simulink model "deliverable2"  (R2020a)
settings: Solver=FixedStepAuto  StartTime=0.0  StopTime=10.0  FixedStep=1e-3  RelTol=1e-3  EnableMultiTasking=on
undefined symbols (not defined in the file): A0, A1, D0, D1, D10, D11, D12, D13, D2, D3, D4, D5, D6, D7, D8, D9, PTA0, PTA1, PTA2, PTB2, PTB23, PTB3, PTB9, PTC16, PTC17, PTC2, PTC3, PTC4, PTD0, PTD1, PTD2, PTD3
libraries: frdmk64flib x21, simulink x3, etargetslib x2
settings Model: ExtModeTrigDuration=5  Creator=Abrar Hussain  LastModifiedBy=Nabil
settings SolverCC: AutoInsertRateTranBlk=on
settings OptimizationCC: EnhancedBackFolding=on  PassReuseOutputArgsAs=Individual arguments  ZeroExternalMemoryAtStartup=off  ZeroInternalMemoryAtStartup=off  MaxStackSize=64  OptimizeBlockOrder=speed  DifferentSizesBufferReuse=on  OptimizationCustomize=off  EfficientTunableParamExpr=on
settings DebuggingCC: ParameterTunabilityLossMsg=error
settings HardwareCC: ProdBitPerPointer=32  ProdBitPerSizeT=32  ProdBitPerPtrDiffT=32  ProdLargestAtomicInteger=Long  ProdLargestAtomicFloat=Double  ProdWordSize=32  ProdHWDeviceType=ARM Compatible->ARM Cortex
settings SFSimCC: MATLABDynamicMemAlloc=off
settings RTWCC: SystemTargetFile=ert.tlc  HardwareBoard=NXP FRDM-K64F  TemplateMakefile=ert_default_tmf  Toolchain=GNU Tools for ARM Embedded Processors
settings CodeAppCC: ForceParamTrailComments=on  IgnoreCustomStorageClasses=off  OperatorAnnotations=on  SimulinkDataObjDesc=on  SFDataObjDesc=on  InsertBlockDesc=on

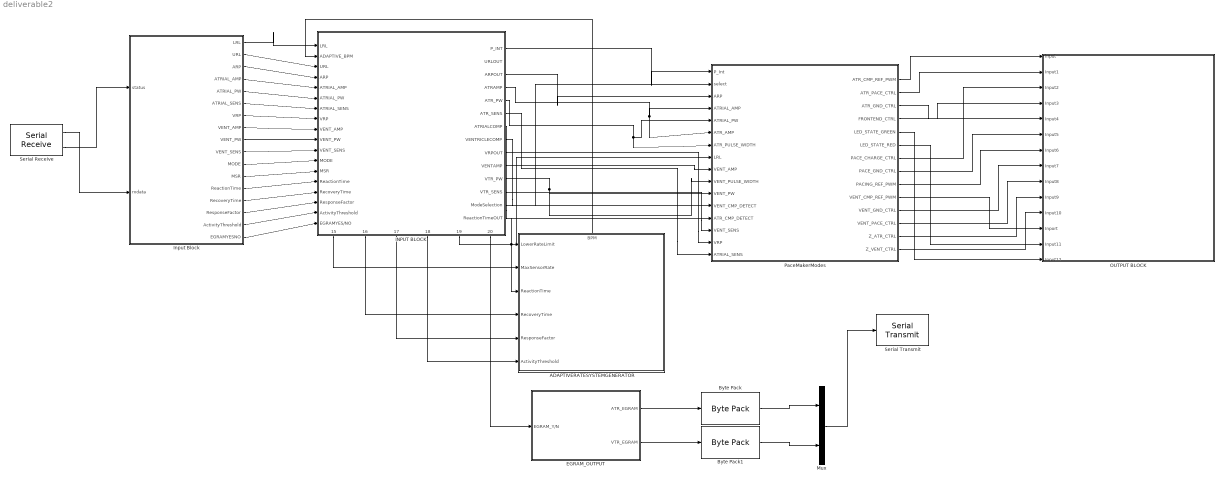
== system deliverable2 ==
  ADAPTIVERATESYSTEMGENERATOR : Subsystem
      settings: PortSchema="{\"entries\":[{\"content\":{\"sides\":[{\"content\":{\"connectorIds\":[\"In1\",\"In2\",\"In3\",\"In4\",\"In5\",\"In6\"]},\"type\":\"ConnectorPlacement.EquallySpacedRectSide\",\"uuid\":\"97e3620a-bd9c-448b-97fc-3b1c936c5d8f\"},{\"content\":{\"connectorIds\":[],\"side\":\"RIGHT\"},\"type\":\"ConnectorPlacement.EquallySpacedRectSide\",\"uuid\":\"57bdd7e3-75eb-4ddf-876e-8d78bd49943e\"},{\"content\":{\"connectorIds\":[\"Out1\"],\"side\":\"TOP\"},\"type\":\"ConnectorPlacement.EquallySpacedRectSide\",\"uuid\":\"a5076879-9988-488c-a84d-5198dc545756\"}]},\"type\":\"ConnectorPlacement.EquallySpacedConnector\",\"uuid\":\"f48a9ccb-b26f-4eb4-a375-26685a890dd7\"}],\"packageUris\":[\"http://schema.mathworks.com/mf0/Connector/19700101\"],\"version\":\"1.0\"}"
  Byte Pack : etargetslib/Byte Pack  datatypes={'double'}  byteAlign=1
  Byte Pack1 : etargetslib/Byte Pack  datatypes={'double'}  byteAlign=1
  EGRAM_OUTPUT : Subsystem
  INPUT BLOCK : Subsystem
      settings: PortSchema="{\"entries\":[{\"content\":{\"sides\":[{\"content\":{\"connectorIds\":[\"In1\",\"In2\",\"In3\",\"In4\",\"In5\",\"In6\",\"In7\",\"In8\",\"In9\",\"In10\",\"In11\",\"In12\",\"In13\",\"In14\",\"In15\",\"In16\",\"In17\",\"In18\"]},\"type\":\"ConnectorPlacement.EquallySpacedRectSide\",\"uuid\":\"b7991482-aae8-494c-b95e-38f3914ca862\"},{\"content\":{\"connectorIds\":[\"Out1\",\"Out2\",\"Out3\",\"Out4\",\"Out5\",\"Out6\",\"Out7\",\"Out8\",\"Out9\",\"Out10\",\"Out11\",\"Out12\",\"Out13\",\"Out14\"],\"side\":\"RIGHT\"},\"type\":\"ConnectorPlacement.EquallySpacedRectSide\",\"uuid\":\"a5db160a-6579-43b0-bce8-09045d3fe5a5\"},{\"content\":{\"connectorIds\":[],\"side\":\"TOP\"},\"type\":\"ConnectorPlacement.EquallySpacedRectSide\",\"uuid\":\"59d47d4e-9fe5-4943-8fba-05eb32ac822f\"},{\"content\":{\"connectorIds\":[\"Out15\",\"Out16\",\"Out17\",\"Out18\",\"Out19\",\"Out20\"],\"side\":\"BOTTOM\"},\"type\":\"ConnectorPlacement.EquallySpacedRectSide\",\"uuid\":\"ee0852ae-153e-4381-9b18-f12d1b0cb66f\"}]},\"type\":\"ConnectorPlacement.EquallySpacedConnector\",\"uuid\":\"9fb077cb-2923-469d-be1e-c13020122ede\"}],\"packageUris\":[\"http://schema.mathworks.com/mf0/Connector/19700101\"],\"version\":\"1.0\"}"
  Input Block : Stateflow chart  TreatAsAtomicUnit=on
  Mux : Mux  Inputs=2
  OUTPUT BLOCK : Subsystem
  PaceMakerModes : Stateflow chart  TreatAsAtomicUnit=on
      settings: PortSchema="{\"entries\":[{\"content\":{\"sides\":[{\"content\":{\"connectorIds\":[\"In1\",\"In2\",\"In3\",\"In4\",\"In5\",\"In6\",\"In7\",\"In8\",\"In9\",\"In10\",\"In11\",\"In12\",\"In13\",\"In14\",\"In15\",\"In16\"]},\"type\":\"ConnectorPlacement.EquallySpacedRectSide\",\"uuid\":\"26878569-42a4-4c6e-8e2e-b0c46cc4aa32\"},{\"content\":{\"connectorIds\":[\"Out1\",\"Out3\",\"Out2\",\"Out4\",\"Out5\",\"Out6\",\"Out7\",\"Out8\",\"Out9\",\"Out10\",\"Out11\",\"Out12\",\"Out13\",\"Out14\"],\"side\":\"RIGHT\"},\"type\":\"ConnectorPlacement.EquallySpacedRectSide\",\"uuid\":\"54e40a9a-b8cb-48bd-a159-657a41086fa1\"},{\"content\":{\"connectorIds\":[],\"side\":\"TOP\"},\"type\":\"ConnectorPlacement.EquallySpacedRectSide\",\"uuid\":\"729d6bf4-f6e0-4315-bd55-b919cf68ae5a\"}]},\"type\":\"ConnectorPlacement.EquallySpacedConnector\",\"uuid\":\"8ffc528b-0e13-4f9b-b36d-bd07e577bd5a\"}],\"packageUris\":[\"http://schema.mathworks.com/mf0/Connector/19700101\"],\"version\":\"1.0\"}"
  Serial Receive : frdmk64flib/Serial Receive  SCIModule=0  Baudrate=uint32(9600)  Parity=None  StopBits=1  HardwareFlowControl=None  ByteOrder=LittleEndian  DataType=uint8  DataLength=20  BlockingMode=off  OutputStatus=on  SampleTime=0.1
  Serial Transmit : frdmk64flib/Serial Transmit  SCIModule=0  Baudrate=uint32(9600)  Parity=None  StopBits=1  HardwareFlowControl=None  ByteOrder=LittleEndian  BlockingMode=on  OutputStatus=off
  wires:
  INPUT BLOCK/20(EGRAMBUTTON) -> EGRAM_OUTPUT/1(EGRAM_Y/N)
  EGRAM_OUTPUT/1(ATR_EGRAM) -> Byte Pack/1
  EGRAM_OUTPUT/2(VTR_EGRAM) -> Byte Pack1/1
  ADAPTIVERATESYSTEMGENERATOR/1(BPM) -> INPUT BLOCK/2(ADAPTIVE_BPM)
  INPUT BLOCK/19(LowerRateLimit) -> PaceMakerModes/8(LRL), ADAPTIVERATESYSTEMGENERATOR/1(LowerRateLimit)
  INPUT BLOCK/15(MaxSensorRate) -> ADAPTIVERATESYSTEMGENERATOR/2(MaxSensorRate)
  INPUT BLOCK/14(ReactionTimeOUT) -> ADAPTIVERATESYSTEMGENERATOR/3(ReactionTime)
  INPUT BLOCK/16(RecoveryTimeOUT) -> ADAPTIVERATESYSTEMGENERATOR/4(RecoveryTime)
  INPUT BLOCK/17(ResponseFactorOUT) -> ADAPTIVERATESYSTEMGENERATOR/5(ResponseFactor)
  INPUT BLOCK/18(ActivityThresholdOUT) -> ADAPTIVERATESYSTEMGENERATOR/6(ActivityThreshold)
  INPUT BLOCK/1(P_INT) -> PaceMakerModes/1(P_Int)
  INPUT BLOCK/3(ARPOUT) -> PaceMakerModes/3(ARP)
  INPUT BLOCK/13(ModeSelection) -> PaceMakerModes/2(select)
  INPUT BLOCK/4(ATRAMP) -> PaceMakerModes/6(ATR_AMP), PaceMakerModes/4(ATRIAL_AMP)
  INPUT BLOCK/5(ATR_PW) -> PaceMakerModes/7(ATR_PULSE_WIDTH), PaceMakerModes/5(ATRIAL_PW)
  INPUT BLOCK/6(ATR_SENS) -> PaceMakerModes/16(ATRIAL_SENS)
  INPUT BLOCK/7(ATRIALCOMP) -> PaceMakerModes/13(ATR_CMP_DETECT)
  INPUT BLOCK/8(VENTRICLECOMP) -> PaceMakerModes/12(VENT_CMP_DETECT)
  INPUT BLOCK/9(VRPOUT) -> PaceMakerModes/15(VRP)
  INPUT BLOCK/10(VENTAMP) -> PaceMakerModes/9(VENT_AMP)
  INPUT BLOCK/11(VTR_PW) -> PaceMakerModes/10(VENT_PULSE_WIDTH), PaceMakerModes/11(VENT_PW)
  INPUT BLOCK/12(VTR_SENS) -> PaceMakerModes/14(VENT_SENS)
  PaceMakerModes/1(ATR_CMP_REF_PWM) -> OUTPUT BLOCK/1(Input)
  PaceMakerModes/3(ATR_PACE_CTRL) -> OUTPUT BLOCK/2(Input1)
  PaceMakerModes/7(PACE_CHARGE_CTRL) -> OUTPUT BLOCK/3(Input2)
  PaceMakerModes/4(FRONTEND_CTRL) -> OUTPUT BLOCK/4(Input3)
  PaceMakerModes/2(ATR_GND_CTRL) -> OUTPUT BLOCK/5(Input4)
  PaceMakerModes/8(PACE_GND_CTRL) -> OUTPUT BLOCK/6(Input5)
  PaceMakerModes/9(PACING_REF_PWM) -> OUTPUT BLOCK/7(Input6)
  PaceMakerModes/14(Z_VENT_CTRL) -> OUTPUT BLOCK/11(Input10)
  PaceMakerModes/13(Z_ATR_CTRL) -> OUTPUT BLOCK/10(Input9)
  PaceMakerModes/12(VENT_PACE_CTRL) -> OUTPUT BLOCK/9(Input8)
  PaceMakerModes/11(VENT_GND_CTRL) -> OUTPUT BLOCK/8(Input7)
  PaceMakerModes/10(VENT_CMP_REF_PWM) -> OUTPUT BLOCK/12(Inport)
  PaceMakerModes/6(LED_STATE_RED) -> OUTPUT BLOCK/13(Input11)
  PaceMakerModes/5(LED_STATE_GREEN) -> OUTPUT BLOCK/14(Input12)
  Input Block/1(LRL) -> INPUT BLOCK/1("LRL ")
  Input Block/2(URL) -> INPUT BLOCK/3(URL)
  Input Block/3(ARP) -> INPUT BLOCK/4(ARP)
  Input Block/4(ATRIAL_AMP) -> INPUT BLOCK/5(ATRIAL_AMP)
  Input Block/5(ATRIAL_PW) -> INPUT BLOCK/6(ATRIAL_PW)
  Input Block/6(ATRIAL_SENS) -> INPUT BLOCK/7(ATRIAL_SENS)
  Input Block/7(VRP) -> INPUT BLOCK/8(VRP)
  Input Block/8(VENT_AMP) -> INPUT BLOCK/9(VENT_AMP)
  Input Block/9(VENT_PW) -> INPUT BLOCK/10(VENT_PW)
  Input Block/10(VENT_SENS) -> INPUT BLOCK/11(VENT_SENS)
  Input Block/11(MODE) -> INPUT BLOCK/12(MODE)
  Input Block/12(MSR) -> INPUT BLOCK/13(MSR)
  Input Block/13(ReactionTime) -> INPUT BLOCK/14(ReactionTime)
  Input Block/14(RecoveryTime) -> INPUT BLOCK/15(RecoveryTime)
  Input Block/15(ResponseFactor) -> INPUT BLOCK/16(ResponseFactor)
  Input Block/16(ActivityThreshold) -> INPUT BLOCK/17(ActivityThreshold)
  Input Block/17(EGRAMYESNO) -> INPUT BLOCK/18(EGRAMYES/NO)
  Serial Receive/2 -> Input Block/1(status)
  Serial Receive/1 -> Input Block/2(rxdata)
  Byte Pack/1 -> Mux/1
  Byte Pack1/1 -> Mux/2
  Mux/1 -> Serial Transmit/1

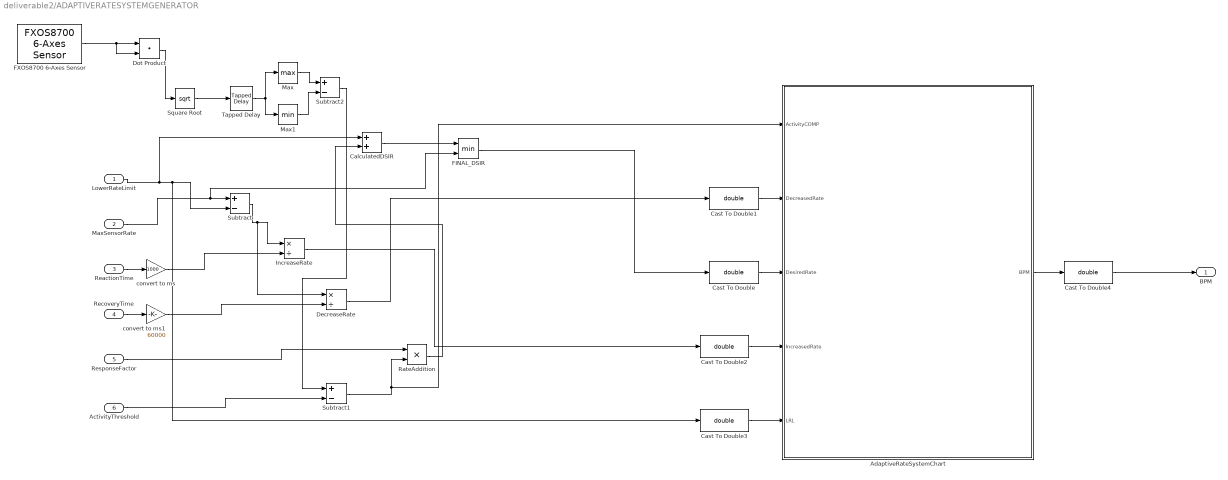
== system deliverable2/ADAPTIVERATESYSTEMGENERATOR ==
  LowerRateLimit : Inport
  MaxSensorRate : Inport  Port=2
  ReactionTime : Inport  Port=3
  RecoveryTime : Inport  Port=4
  ResponseFactor : Inport  Port=5
  ActivityThreshold : Inport  Port=6
  AdaptiveRateSystemChart : Stateflow chart  TreatAsAtomicUnit=on
  CalculatedDSIR : Sum
  Cast To Double{,1..4} (5 alike) : DataTypeConversion  OutDataTypeStr=double
  DecreaseRate : Product  Inputs=*/
  Dot Product : DotProduct  RndMeth=Nearest  InputSameDT=on  OutDataTypeStr=Inherit: Inherit via internal rule
  FINAL_DSIR : MinMax  Inputs=2
  FXOS8700 6-Axes Sensor : frdmk64flib/FXOS8700 6-Axes Sensor  Activesensor=Accelerometer only  ODR=800Hz  HybridODR=400Hz  Accelfullrange=-4g to +4g  SampleTime=-1
  IncreaseRate : Product  Inputs=*/
  Max : MinMax  Function=max
  Max1 : MinMax
  RateAddition : Product
  Square Root : Sqrt  SaturateOnIntegerOverflow=on
  Subtract : Sum  Inputs=+-
  Subtract1 : Sum  Inputs=+-
  Subtract2 : Sum  Inputs=+-
  Tapped Delay : simulink/Discrete/Tapped Delay  vinit=0.0  samptime=0.002  NumDelays=99  DelayOrder=Oldest  includeCurrent=on
  convert to ms : Gain  Gain=1000
  convert to ms1 : Gain  Gain=60000
  BPM : Outport
  wires:
  LowerRateLimit/1 -> CalculatedDSIR/1, Cast To Double3/1, Subtract/2
  Subtract/1 -> DecreaseRate/1, IncreaseRate/1
  ReactionTime/1 -> convert to ms/1
  RecoveryTime/1 -> convert to ms1/1
  ActivityThreshold/1 -> Subtract1/2
  Subtract2/1 -> Subtract1/1
  ResponseFactor/1 -> RateAddition/1
  RateAddition/1 -> CalculatedDSIR/2
  CalculatedDSIR/1 -> FINAL_DSIR/1
  MaxSensorRate/1 -> FINAL_DSIR/2, Subtract/1
  FINAL_DSIR/1 -> Cast To Double/1
  IncreaseRate/1 -> Cast To Double2/1
  DecreaseRate/1 -> Cast To Double1/1
  AdaptiveRateSystemChart/1(BPM) -> Cast To Double4/1
  Subtract1/1 -> AdaptiveRateSystemChart/1(ActivityCOMP), RateAddition/2
  Cast To Double1/1 -> AdaptiveRateSystemChart/2(DecreasedRate)
  Cast To Double/1 -> AdaptiveRateSystemChart/3(DesiredRate)
  Cast To Double2/1 -> AdaptiveRateSystemChart/4(IncreasedRate)
  Cast To Double3/1 -> AdaptiveRateSystemChart/5(LRL)
  Cast To Double4/1 -> BPM/1
  convert to ms/1 -> IncreaseRate/2
  convert to ms1/1 -> DecreaseRate/2
  Tapped Delay/1 -> Max/1, Max1/1
  Max1/1 -> Subtract2/2
  FXOS8700 6-Axes Sensor/1 -> Dot Product/2, Dot Product/1
  Max/1 -> Subtract2/1
  Square Root/1 -> Tapped Delay/1
  Dot Product/1 -> Square Root/1

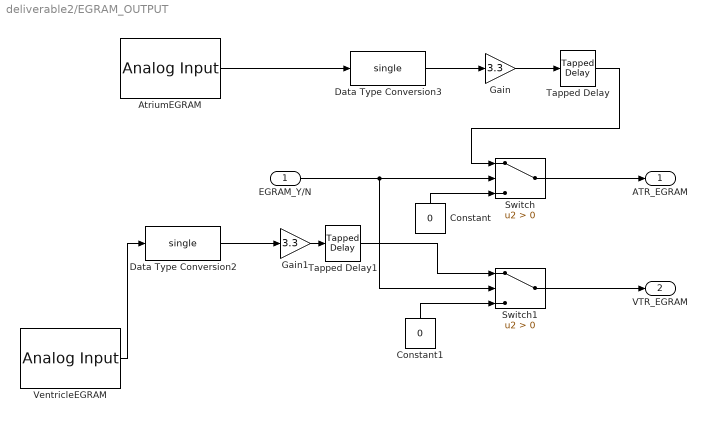
== system deliverable2/EGRAM_OUTPUT ==
  EGRAM_Y/N : Inport
  AtriumEGRAM : frdmk64flib/Analog Input  Whichpin=PTB2 (A0)  SampleTime=-1
  Constant : Constant  Value=0
  Constant1 : Constant  Value=0
  Data Type Conversion2 : DataTypeConversion  OutDataTypeStr=single  RndMeth=Nearest
  Data Type Conversion3 : DataTypeConversion  OutDataTypeStr=single  RndMeth=Nearest
  Gain : Gain  Gain=3.3
  Gain1 : Gain  Gain=3.3
  Switch : Switch  Criteria=u2 > Threshold
  Switch1 : Switch  Criteria=u2 > Threshold
  Tapped Delay : simulink/Discrete/Tapped Delay  vinit=0.0  samptime=0.002  NumDelays=9  DelayOrder=Oldest  includeCurrent=on
  Tapped Delay1 : simulink/Discrete/Tapped Delay  vinit=0.0  samptime=0.002  NumDelays=9  DelayOrder=Oldest  includeCurrent=on
  VentricleEGRAM : frdmk64flib/Analog Input  Whichpin=PTB3 (A1)  SampleTime=-1
  ATR_EGRAM : Outport
  VTR_EGRAM : Outport  Port=2
  wires:
  EGRAM_Y/N/1 -> Switch1/2, Switch/2
  Switch/1 -> ATR_EGRAM/1
  Switch1/1 -> VTR_EGRAM/1
  Data Type Conversion3/1 -> Gain/1
  Gain1/1 -> Tapped Delay1/1
  VentricleEGRAM/1 -> Data Type Conversion2/1
  Tapped Delay1/1 -> Switch1/1
  Tapped Delay/1 -> Switch/1
  AtriumEGRAM/1 -> Data Type Conversion3/1
  Gain/1 -> Tapped Delay/1
  Data Type Conversion2/1 -> Gain1/1
  Constant/1 -> Switch/3
  Constant1/1 -> Switch1/3

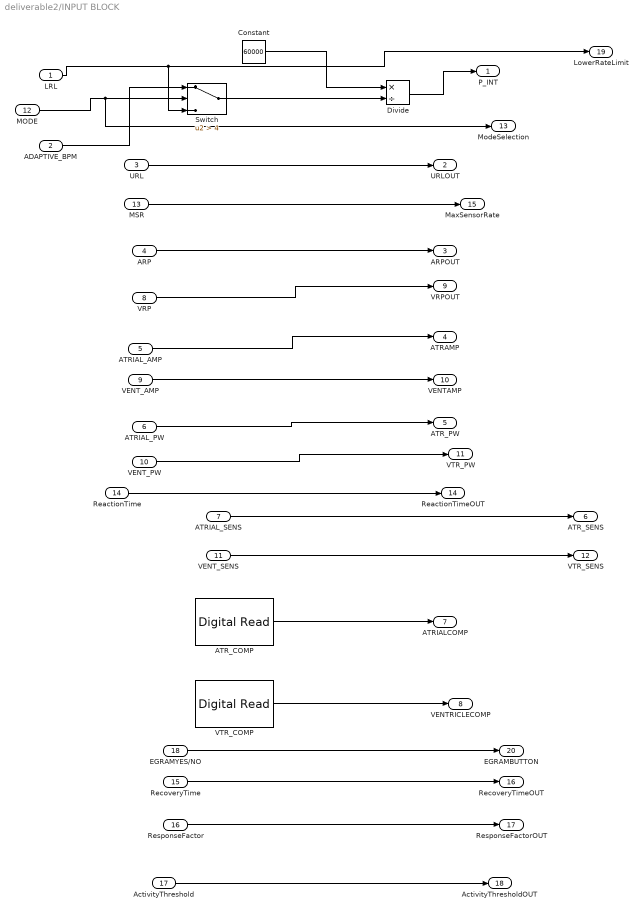
== system deliverable2/INPUT BLOCK ==
  "LRL " : Inport
  ADAPTIVE_BPM : Inport  Port=2
  URL : Inport  Port=3
  ARP : Inport  Port=4
  ATRIAL_AMP : Inport  Port=5
  ATRIAL_PW : Inport  Port=6
  ATRIAL_SENS : Inport  Port=7
  VRP : Inport  Port=8
  VENT_AMP : Inport  Port=9
  VENT_PW : Inport  Port=10
  VENT_SENS : Inport  Port=11
  MODE : Inport  Port=12
  MSR : Inport  Port=13
  ReactionTime : Inport  Port=14
  RecoveryTime : Inport  Port=15
  ResponseFactor : Inport  Port=16
  ActivityThreshold : Inport  Port=17
  EGRAMYES/NO : Inport  Port=18
  ATR_COMP : frdmk64flib/Digital Read  Whichpin=PTC16 (D0)  SampleTime=-1
  Constant : Constant  Value=60000
  Divide : Product  Inputs=*/
  Switch : Switch  Criteria=u2 > Threshold  Threshold=4
  VTR_COMP : frdmk64flib/Digital Read  Whichpin=PTC17 (D1)  SampleTime=-1
  P_INT : Outport
  URLOUT : Outport  Port=2
  ARPOUT : Outport  Port=3
  ATRAMP : Outport  Port=4
  ATR_PW : Outport  Port=5
  ATR_SENS : Outport  Port=6
  ATRIALCOMP : Outport  Port=7
  VENTRICLECOMP : Outport  Port=8
  VRPOUT : Outport  Port=9
  VENTAMP : Outport  Port=10
  VTR_PW : Outport  Port=11
  VTR_SENS : Outport  Port=12
  ModeSelection : Outport  Port=13
  ReactionTimeOUT : Outport  Port=14
  MaxSensorRate : Outport  Port=15
  RecoveryTimeOUT : Outport  Port=16
  ResponseFactorOUT : Outport  Port=17
  ActivityThresholdOUT : Outport  Port=18
  LowerRateLimit : Outport  Port=19
  EGRAMBUTTON : Outport  Port=20
  wires:
  URL/1 -> URLOUT/1
  ARP/1 -> ARPOUT/1
  ATR_COMP/1 -> ATRIALCOMP/1
  ATRIAL_AMP/1 -> ATRAMP/1
  ATRIAL_PW/1 -> ATR_PW/1
  ATRIAL_SENS/1 -> ATR_SENS/1
  Constant/1 -> Divide/1
  Divide/1 -> P_INT/1
  Switch/1 -> Divide/2
  "LRL "/1 -> LowerRateLimit/1, Switch/3
  ADAPTIVE_BPM/1 -> Switch/1
  VTR_COMP/1 -> VENTRICLECOMP/1
  VRP/1 -> VRPOUT/1
  VENT_AMP/1 -> VENTAMP/1
  VENT_PW/1 -> VTR_PW/1
  VENT_SENS/1 -> VTR_SENS/1
  MODE/1 -> ModeSelection/1, Switch/2
  MSR/1 -> MaxSensorRate/1
  ReactionTime/1 -> ReactionTimeOUT/1
  RecoveryTime/1 -> RecoveryTimeOUT/1
  ResponseFactor/1 -> ResponseFactorOUT/1
  ActivityThreshold/1 -> ActivityThresholdOUT/1
  EGRAMYES/NO/1 -> EGRAMBUTTON/1

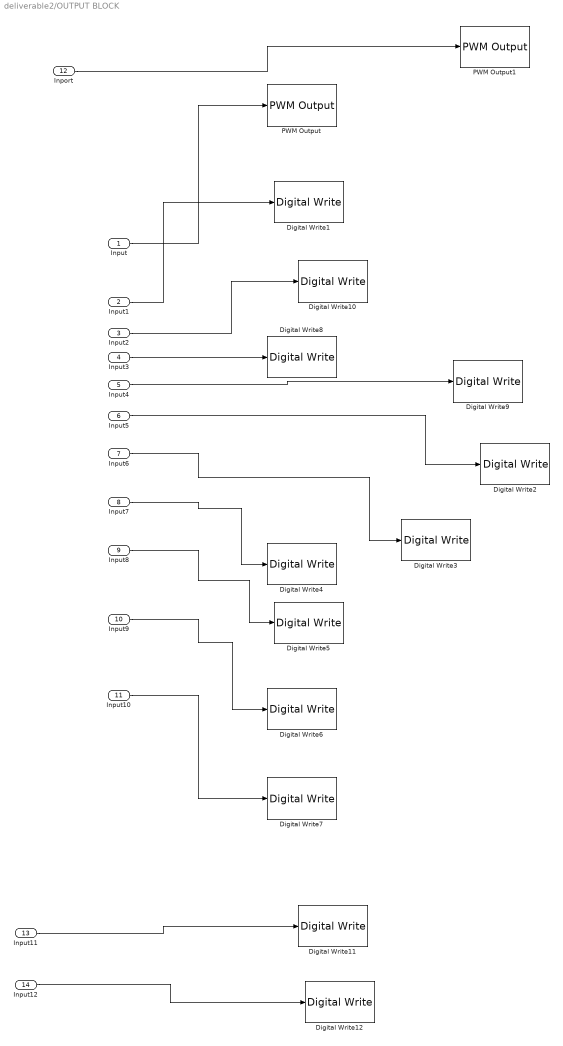
== system deliverable2/OUTPUT BLOCK ==
  Input : Inport
  Input1 : Inport  Port=2
  Input2 : Inport  Port=3
  Input3 : Inport  Port=4
  Input4 : Inport  Port=5
  Input5 : Inport  Port=6
  Input6 : Inport  Port=7
  Input7 : Inport  Port=8
  Input8 : Inport  Port=9
  Input9 : Inport  Port=10
  Input10 : Inport  Port=11
  Inport : Inport  Port=12
  Input11 : Inport  Port=13
  Input12 : Inport  Port=14
  Digital Write1 : frdmk64flib/Digital Write  Whichpin=PTA0 (D8)
  Digital Write10 : frdmk64flib/Digital Write  Whichpin=PTB9 (D2)
  Digital Write11 : frdmk64flib/Digital Write  Whichpin=RED_LED
  Digital Write12 : frdmk64flib/Digital Write  Whichpin=GREEN_LED
  Digital Write2 : frdmk64flib/Digital Write  Whichpin=PTD0 (D10)
  Digital Write3 : frdmk64flib/Digital Write  Whichpin=PTA2 (D5)
  Digital Write4 : frdmk64flib/Digital Write  Whichpin=PTD3 (D12)
  Digital Write5 : frdmk64flib/Digital Write  Whichpin=PTC4 (D9)
  Digital Write6 : frdmk64flib/Digital Write  Whichpin=PTB23 (D4)
  Digital Write7 : frdmk64flib/Digital Write  Whichpin=PTC3 (D7)
  Digital Write8 : frdmk64flib/Digital Write  Whichpin=PTD1 (D13)
  Digital Write9 : frdmk64flib/Digital Write  Whichpin=PTD2 (D11)
  PWM Output : frdmk64flib/PWM Output  Whichpin=PTC2 (D6)  InitialFrequency=2000  InitialDutyCycle=0
  PWM Output1 : frdmk64flib/PWM Output  Whichpin=PTA1 (D3)  InitialFrequency=2000  InitialDutyCycle=0
  wires:
  Input/1 -> PWM Output/1
  Input1/1 -> Digital Write1/1
  Input10/1 -> Digital Write7/1
  Input9/1 -> Digital Write6/1
  Input8/1 -> Digital Write5/1
  Input7/1 -> Digital Write4/1
  Input6/1 -> Digital Write3/1
  Input5/1 -> Digital Write2/1
  Input4/1 -> Digital Write9/1
  Input3/1 -> Digital Write8/1
  Input2/1 -> Digital Write10/1
  Inport/1 -> PWM Output1/1
  Input11/1 -> Digital Write11/1
  Input12/1 -> Digital Write12/1

== stateflow chart deliverable2/ADAPTIVERATESYSTEMGENERATOR/AdaptiveRateSystemChart ==
  state PowerOnReset
    entry:
    BPM = LRL;
    elapsed_time = 0;
  state ActivityGreaterDecrease
    entry:
    elapsed_time = elapsed(msec);
    BPM = BPM - (DecreasedRate*elapsed_time);
  state ActivitySmallerDecrease
    entry:
    elapsed_time = elapsed(msec);
    BPM = BPM - (DecreasedRate*elapsed_time);
  state CheckActivity
  state ActivityGreaterIncrease
    entry:
    elapsed_time = elapsed(msec);
    BPM = BPM + (IncreasedRate*elapsed_time);
  state DesiredRateMet
    entry:
    elapsed_time = 0;
    BPM = DesiredRate;
  state LowerRateMet
    entry:
    BPM = LRL;
    elapsed_time = 0;
  (default) -> PowerOnReset
  PowerOnReset -> CheckActivity
  (junction 13) -> ActivityGreaterDecrease [order 1] : [DesiredRate < BPM]
  ActivityGreaterDecrease -> DesiredRateMet : [BPM <= DesiredRate]
  CheckActivity -> (junction 13) [order 1] : [ActivityCOMP  > 0]
  CheckActivity -> (junction 30) [order 2] : [ActivityCOMP <= 0]
  (junction 13) -> ActivityGreaterIncrease [order 2] : [DesiredRate > BPM]
  (junction 13) -> DesiredRateMet [order 3] : [BPM == DesiredRate]
  (junction 30) -> ActivitySmallerDecrease [order 2] : [BPM  >= LRL]
  (junction 30) -> LowerRateMet [order 1] : [BPM == LRL]
  (junction 27) -> CheckActivity : [after(60/BPM,sec)]
  ActivitySmallerDecrease -> LowerRateMet : [BPM <= LRL]
  DesiredRateMet -> (junction 27)
  LowerRateMet -> (junction 27)
  ActivityGreaterIncrease -> DesiredRateMet : [BPM >= DesiredRate]
  data: BPM output; ActivityCOMP input; DecreasedRate input; DesiredRate input; IncreasedRate input; LRL input; elapsed_time local

== stateflow chart deliverable2/Input Block ==
  state Set_param
    entry:
    LRL = cast(rxdata(3),'uint16');
    URL = cast(rxdata(4),'uint16');
    ARP = cast(rxdata(5),'uint16');
    ATRIAL_AMP = cast(rxdata(6),'double');
    ATRIAL_PW = cast(rxdata(7),'uint16');
    ATRIAL_SENS = cast(rxdata(8),'double');
    VRP = cast(rxdata(9),'uint16');
    VENT_AMP = cast(rxdata(10),'double');
    VENT_PW = cast(rxdata(11),'double');
    VENT_SENS = cast(rxdata(12),'double');
    MODE = cast(rxdata(13),'uint16');
    MSR = cast(rxdata(14),'uint16');
    ReactionTime = cast(rxdata(15),'uint16');
    RecoveryTime = cast(rxdata(16),'uint16');
    ResponseFactor = cast(rxdata(17),'double');
    ActivityThreshold = cast(rxdata(18),'double');
    EGRAMYESNO = cast(rxdata(19),'uint16');
  state Initial
    entry:
    LRL = 60;
    URL = 120;
    ARP = 250;
    ATRIAL_AMP = 3.75;
    ATRIAL_PW = 0;
    ATRIAL_SENS = 0.75;
    VRP = 320;
    VENT_AMP = 3.75;
    VENT_PW = 0;
    VENT_SENS = 2.5;
    MODE = 5;
    MSR = 120;
    ReactionTime = 30;
    RecoveryTime = 5;
    ResponseFactor = 8;
    ActivityThreshold = 30;
    EGRAMYESNO = 0;
  state Standby
    %waiting for COM
  (default) -> Initial
  Set_param -> Standby
  (junction 62) -> ? : [rxdata(2)==hex2dec('00')]
  (junction 65) -> Standby [order 2]
  Standby -> (junction 65) : [status==0]
  (junction 65) -> (junction 62) [order 1]
  Initial -> Standby
  (junction 62) -> ? [commented out] : [rxdata(57)==hex2dec('01')]
  data: LRL output; URL output; ARP output; ATRIAL_AMP output; ATRIAL_PW output; ATRIAL_SENS output; VRP output; VENT_AMP output; VENT_PW output; VENT_SENS output; MODE output; MSR output; ReactionTime output; RecoveryTime output; ResponseFactor output; ActivityThreshold output; EGRAMYESNO output; status input; rxdata input

== stateflow chart deliverable2/PaceMakerModes ==
  note: MODE DIRECTORY
      |
      | 1 - AOO
      |
      | 2 - VOO
      |
      | 3 - AAI
      |
      | 4 - VVI
      |
      | 5 - AOOR
      |
      | 6 - VOOR
      |
      | 7 - AAIR
      |
      | 8 - VVIR
  state AAI
    state C22_Charge_C21_Discharge
      entry:
      FRONTEND_CTRL = 1; %sensing ON
      %C22 Charge
      VENT_PACE_CTRL = 0;
      ATR_PACE_CTRL = 0;
      PACING_REF_PWM = ATRIAL_AMP;
      PACE_CHARGE_CTRL = 1;
      %We can also discharge C21 from previous pacing
      PACE_GND_CTRL = 1;
      ATR_PACE_CTRL = 0;
      Z_VENT_CTRL = 0;
      Z_ATR_CTRL = 0;
      VENT_PACE_CTRL = 0;
      VENT_GND_CTRL = 0;
      ATR_GND_CTRL = 1;
      ATR_CMP_REF_PWM = ATRIAL_SENS;
    state Pacing
      entry:
      %sensing off
      FRONTEND_CTRL = 0;
      %PACE
      PACE_CHARGE_CTRL = 0;
      PACE_GND_CTRL = 1;
      VENT_PACE_CTRL = 0;
      VENT_GND_CTRL = 0;
      Z_VENT_CTRL = 0;
      Z_ATR_CTRL = 0;
      ATR_GND_CTRL = 0;
      ATR_PACE_CTRL = 1;
      PACING_REF_PWM = ATRIAL_AMP;
    state ARP_Period
      entry:
      FRONTEND_CTRL = 0; % No sensing
      ATR_PACE_CTRL = 0;
      VENT_PACE_CTRL = 0;
      ATR_GND_CTRL = 1;
      PACE_CHARGE_CTRL = 0;
      PACE_GND_CTRL = 1;
      PACING_REF_PWM = ATRIAL_AMP;
    (junction 7) -> AAI.Pacing [order 1] : [(ATR_CMP_DETECT == false ) && after(P_Int - ATRIAL_PW - ARP,msec)]
    C22_Charge_C21_Discharge -> (junction 7)
    (default) -> C22_Charge_C21_Discharge
    (junction 7) -> ARP_Period [order 2] : [ATR_CMP_DETECT == true]
    ARP_Period -> C22_Charge_C21_Discharge : after(ARP,msec)
    AAI.Pacing -> ARP_Period : after(ATRIAL_PW, msec)
  state VVI
    state Pacing
      entry:
      %sensing off
      FRONTEND_CTRL = 0;
      %PACE
      PACE_CHARGE_CTRL = 0;
      PACE_GND_CTRL = 1;
      VENT_PACE_CTRL = 1;
      VENT_GND_CTRL = 0;
      Z_VENT_CTRL = 0;
      Z_ATR_CTRL = 0;
      ATR_GND_CTRL = 0;
      ATR_PACE_CTRL = 0;
      PACING_REF_PWM = VENT_AMP;
    state VRP_CHARING %C22_Charge_C21_Discharge
      entry:
      FRONTEND_CTRL = 1; %sensing ON
      %C22 Charge
      VENT_PACE_CTRL = 0;
      ATR_PACE_CTRL = 0;
      PACING_REF_PWM = VENT_AMP;
      PACE_CHARGE_CTRL = 1;
      %We can also discharge C21 from previous pacing
      PACE_GND_CTRL = 1;
      ATR_PACE_CTRL = 0;
      Z_VENT_CTRL = 0;
      Z_ATR_CTRL = 0;
      VENT_PACE_CTRL = 0;
      VENT_GND_CTRL = 1;
      ATR_GND_CTRL = 0;
      VENT_CMP_REF_PWM = VENT_SENS;
    state VRP_Period
      entry:
      FRONTEND_CTRL = 0; % No sensing
      ATR_PACE_CTRL = 0;
      VENT_PACE_CTRL = 0;
      VENT_GND_CTRL = 1;
      PACE_CHARGE_CTRL = 0;
      PACE_GND_CTRL = 1;
      PACING_REF_PWM = VENT_AMP;
    (default) -> VRP_CHARING %C22_Charge_C21_Discharge
    VRP_CHARING %C22_Charge_C21_Discharge -> (junction 39)
    (junction 39) -> VVI.Pacing [order 1] : [(VENT_CMP_DETECT == false ) && after(P_Int - VENT_PW - VRP,msec)]
    (junction 39) -> VRP_Period [order 2] : [VENT_CMP_DETECT == true]
    VRP_Period -> VRP_CHARING %C22_Charge_C21_Discharge : after(VRP,msec)
    VVI.Pacing -> VRP_Period : after(VENT_PW, msec)
  state ModeSelection
  state VOO
    state VOO_INTERVAL_TIMER
      entry:
      VENT_PACE_CTRL = 0;
      PACE_CHARGE_CTRL = 1;
      PACING_REF_PWM = VENT_AMP;
      VENT_GND_CTRL = 1;
      PACE_GND_CTRL = 1;
      ATR_PACE_CTRL = 0;
      ATR_GND_CTRL = 0;
      Z_VENT_CTRL = 0;
      LED_STATE_RED=true;
      LED_STATE_GREEN=false;
    state VOO_PACE_DELIVERY
      entry:
      VENT_PACE_CTRL = 1;
      PACE_CHARGE_CTRL = 0;
      VENT_GND_CTRL = 0;
      PACE_GND_CTRL = 1;
      ATR_PACE_CTRL = 0;
      ATR_GND_CTRL = 0;
      Z_VENT_CTRL = 0;
      LED_STATE_RED=false;
      LED_STATE_GREEN=true;
    VOO_INTERVAL_TIMER -> VOO_PACE_DELIVERY : [after(P_Int-VENT_PULSE_WIDTH,msec)]
    VOO_PACE_DELIVERY -> VOO_INTERVAL_TIMER : [after(VENT_PULSE_WIDTH,msec)]
    (default) -> VOO_INTERVAL_TIMER
  state AOO
    state AOO_INTERVAL_TIMER
      entry:
      ATR_PACE_CTRL = 0;
      PACE_CHARGE_CTRL = 1;
      PACING_REF_PWM = ATR_AMP;
      ATR_GND_CTRL = 1;
      PACE_GND_CTRL = 1;
      VENT_PACE_CTRL = 0;
      VENT_GND_CTRL = 0;
      Z_ATR_CTRL = 0;
      LED_STATE_RED=true;
      LED_STATE_GREEN=false;
    state AOO_PACE_DELIVERY
      entry:
      ATR_PACE_CTRL = 1;
      PACE_CHARGE_CTRL = 0;
      ATR_GND_CTRL = 0;
      PACE_GND_CTRL = 1;
      VENT_PACE_CTRL = 0;
      VENT_GND_CTRL = 0;
      Z_VENT_CTRL = 0;
      LED_STATE_RED=false;
      LED_STATE_GREEN=true;
    AOO_INTERVAL_TIMER -> AOO_PACE_DELIVERY : [after(P_Int-ATR_PULSE_WIDTH,msec)]
    AOO_PACE_DELIVERY -> AOO_INTERVAL_TIMER : [after(ATR_PULSE_WIDTH,msec)]
    (default) -> AOO_INTERVAL_TIMER
  ModeSelection -> AAI [order 1] : [select == 3 || select == 7]
  ModeSelection -> VVI [order 2] : [select == 4 || select == 8 ]
  (default) -> ModeSelection
  AAI -> ModeSelection : [select ~= 3 && select ~= 7]
  VVI -> ModeSelection : [select ~= 4 && select ~=8]
  ModeSelection -> AOO [order 3] : [select == 1 || select == 5]
  VOO -> ModeSelection : [select ~= 2 && select ~= 6]
  ModeSelection -> VOO [order 4] : [select == 2 || select == 6]
  AOO -> ModeSelection : [select ~= 1 && select ~= 5]
  data: P_Int input; select input; ATR_CMP_REF_PWM output; ATR_GND_CTRL output; ATR_PACE_CTRL output; FRONTEND_CTRL output; LED_STATE_GREEN output; LED_STATE_RED output; PACE_CHARGE_CTRL output; PACE_GND_CTRL output; PACING_REF_PWM output; VENT_CMP_REF_PWM output; VENT_GND_CTRL output; VENT_PACE_CTRL output; Z_ATR_CTRL output; Z_VENT_CTRL output; ARP input; ATRIAL_AMP input; ATRIAL_PW input; ATR_AMP input; ATR_PULSE_WIDTH input; LRL input; VENT_AMP input; VENT_PULSE_WIDTH input; VENT_PW input; VENT_CMP_DETECT input; ATR_CMP_DETECT input; VENT_SENS input; VRP input; ATRIAL_SENS input
